simulink model "Controllore"  (R2024b)
settings: Solver=VariableStepAuto  StartTime=0.0  StopTime=10  RelTol=1e-3
undefined symbols (not defined in the file or in its folder): dcvolt, ia_limite, kamp, kdt, ki, klim, kp, kt, kv, V_kp, Vnom
libraries: cstblocks x2
settings Model: Creator=turco  LastModifiedBy=turco

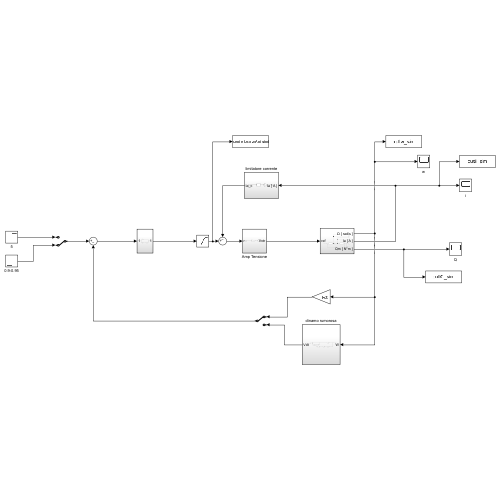
[thumbnail: Simulink's stored preview of the top-level diagram]
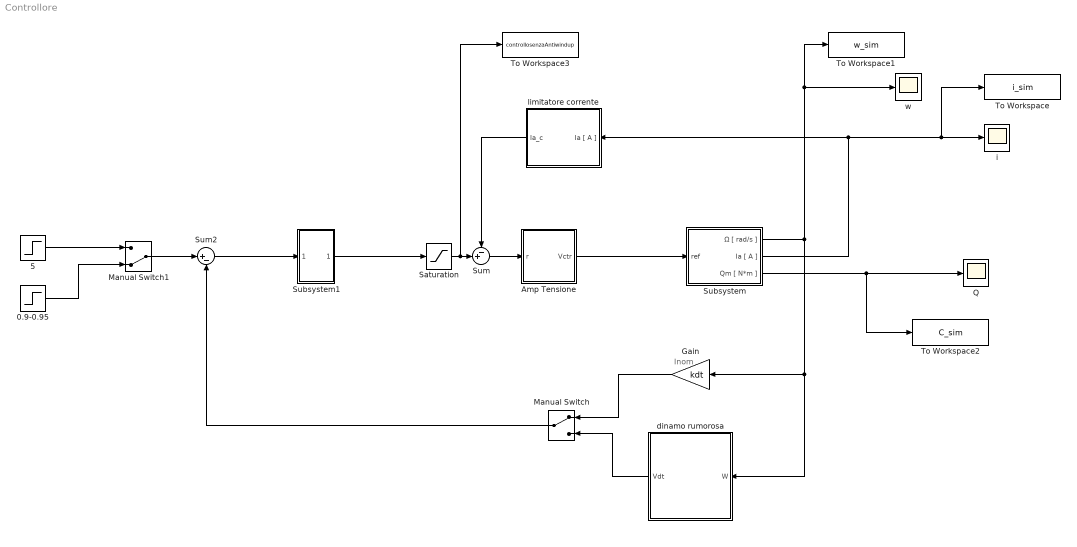
== system Controllore ==
  note: Inom
  0.9-0.95 : Step  Time=5  Before=V_kp  After=V_kp+0.05  SampleTime=0
  5 : Step  After=5  SampleTime=0
  Amp Tensione : Subsystem
  Gain : Gain  Gain=kdt
  Manual Switch : ManualSwitch
  Manual Switch1 : ManualSwitch  CurrentSetting=0
  Q : Scope
  Saturation : Saturate  UpperLimit=5  LowerLimit=-5
  Subsystem : Subsystem
  Subsystem1 : Subsystem
  Sum : Sum  Inputs=-+|
  Sum2 : Sum  Inputs=|+-
  To Workspace : ToWorkspace  VariableName=i_sim  SaveFormat=Timeseries  SampleTime=-1
  To Workspace1 : ToWorkspace  VariableName=w_sim  SaveFormat=Timeseries  SampleTime=-1
  To Workspace2 : ToWorkspace  VariableName=C_sim  SaveFormat=Timeseries  SampleTime=-1
  To Workspace3 : ToWorkspace  VariableName=controllosenzaAntiwindup  SaveFormat=Timeseries  SampleTime=-1
  dinamo rumorosa : Subsystem
  i : Scope
  limitatore corrente : Subsystem
  w : Scope
  wires:
  limitatore corrente/1(Ia_c) -> Sum/1
  Subsystem/3(Qm [ N*m ]) -> To Workspace2/1, Q/1
  Subsystem/1(Ω [ rad/s ]) -> To Workspace1/1, w/1, dinamo rumorosa/1(W), Gain/1
  Sum/1 -> Amp Tensione/1(r)
  Gain/1 -> Manual Switch/1
  Subsystem/2(Ia [ A ]) -> To Workspace/1, i/1, limitatore corrente/1(Ia [ A ])
  Amp Tensione/1(Vctr) -> Subsystem/1(ref)
  Saturation/1 -> To Workspace3/1, Sum/2
  Manual Switch/1 -> Sum2/2
  dinamo rumorosa/1(Vdt) -> Manual Switch/2
  Sum2/1 -> Subsystem1/1(In1)
  Subsystem1/1(Out1) -> Saturation/1
  0.9-0.95/1 -> Manual Switch1/2
  5/1 -> Manual Switch1/1
  Manual Switch1/1 -> Sum2/1

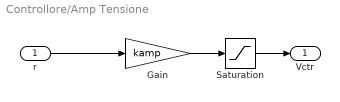
== system Controllore/Amp Tensione ==
  r : Inport
  Gain : Gain  Gain=kamp
  Saturation : Saturate  UpperLimit=+Vnom*1.2  LowerLimit=-Vnom*1.2
  Vctr : Outport
  wires:
  r/1 -> Gain/1
  Saturation/1 -> Vctr/1
  Gain/1 -> Saturation/1

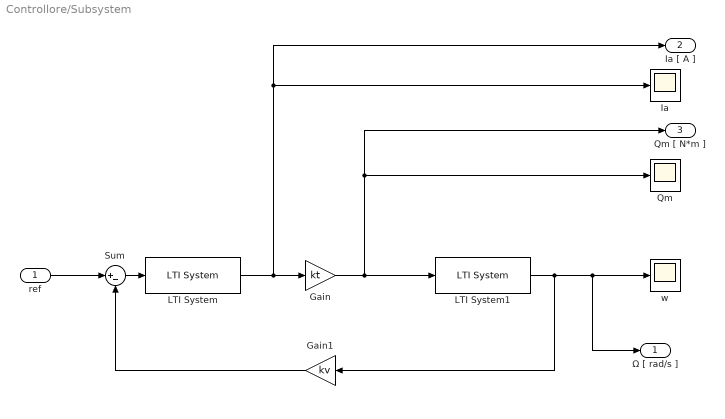
== system Controllore/Subsystem ==
  ref : Inport
  Gain : Gain  Gain=kt
  Gain1 : Gain  Gain=kv
  Ia : Scope
  LTI System : cstblocks/LTI System  sys=Pel  IC=[]  PadeOrder=0
  LTI System1 : cstblocks/LTI System  sys=Pmec  IC=[]  PadeOrder=0
  "Qm " : Scope
  Sum : Sum  Inputs=|+-
  w : Scope
  Ω [ rad/s ] : Outport
  Ia [ A ] : Outport  Port=2
  Qm [ N*m ] : Outport  Port=3
  wires:
  LTI System1/1 -> Ω [ rad/s ]/1, w/1, Gain1/1
  Gain1/1 -> Sum/2
  Gain/1 -> Qm [ N*m ]/1, "Qm "/1, LTI System1/1
  Sum/1 -> LTI System/1
  LTI System/1 -> Ia [ A ]/1, Ia/1, Gain/1
  ref/1 -> Sum/1

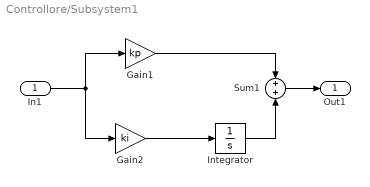
== system Controllore/Subsystem1 ==
  In1 : Inport
  Gain1 : Gain  Gain=kp
  Gain2 : Gain  Gain=ki
  Integrator : Integrator  UpperSaturationLimit=+dcvolt  LowerSaturationLimit=-dcvolt
  Sum1 : Sum
  Out1 : Outport
  wires:
  Integrator/1 -> Sum1/2
  In1/1 -> Gain2/1, Gain1/1
  Sum1/1 -> Out1/1
  Gain1/1 -> Sum1/1
  Gain2/1 -> Integrator/1

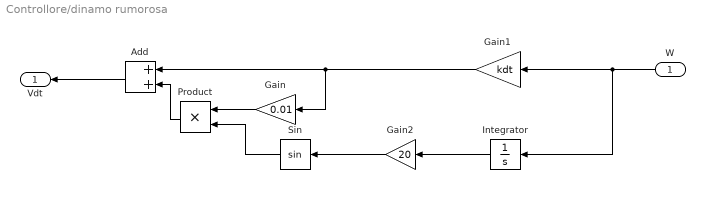
== system Controllore/dinamo rumorosa ==
  W : Inport
  Add : Sum
  Gain : Gain  Gain=0.01
  Gain1 : Gain  Gain=kdt
  Gain2 : Gain  Gain=20
  Integrator : Integrator
  Product : Product
  Sin : Trigonometry
  Vdt : Outport
  wires:
  Product/1 -> Add/2
  W/1 -> Gain1/1, Integrator/1
  Sin/1 -> Product/2
  Gain1/1 -> Add/1, Gain/1
  Add/1 -> Vdt/1
  Integrator/1 -> Gain2/1
  Gain2/1 -> Sin/1
  Gain/1 -> Product/1

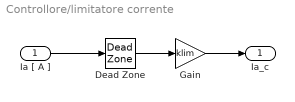
== system Controllore/limitatore corrente ==
  Ia [ A ] : Inport
  Dead Zone : DeadZone  LowerValue=-ia_limite  UpperValue=+ia_limite
  Gain : Gain  Gain=klim
  Ia_c : Outport
  wires:
  Gain/1 -> Ia_c/1
  Ia [ A ]/1 -> Dead Zone/1
  Dead Zone/1 -> Gain/1
